simulink model "Planta_6_5_24_V2"  (R2021a)
settings: Solver=VariableStepAuto  StartTime=0.0  StopTime=130  FixedStep=0.002  MaxStep=1e-3  RelTol=1e-4
model workspace (MAT data in the model file):
  VelMin = 0.5
  vMax = -0.3
values from neighbouring files (symbols this model uses):
  ax_max = 0.8    [valoresPlanta_29_9_24.m]    (also in valoresPlanta_v4.m)
  ay_max = 0.75    [valoresPlanta_29_9_24.m]    (also in valoresPlanta_v4.m)
  bcy = 1e7    (= 10000000)    [Valores_1.m]    (also in valoresPlanta.m; valoresPlanta_29_9_24.m; valoresPlanta_V3.m; valoresPlanta_v4.m)
  bh_eq = bhm*ih^2+bhd    (= 8720)    [Valores.m]    (also in Valores_1.m; valoresPlanta.m; valoresPlanta_29_9_24.m; valoresPlanta_V3.m)
  bhb = 1e8    (= 100000000)    [Valores.m]    (also in Valores_1.m; valoresPlanta.m; valoresPlanta_29_9_24.m; valoresPlanta_V3.m)
  bhEb = 2.2e9    (= 2200000000)    [Valores.m]    (also in Valores_1.m; valoresPlanta.m; valoresPlanta_29_9_24.m; valoresPlanta_V3.m)
  bt = 90.0    (= 90)    [Valores.m]    (also in Valores_1.m; valoresPlanta.m; valoresPlanta_29_9_24.m; valoresPlanta_V3.m)
  bt_eq = btd+(btm*(it^2))    (= 5401.8)    [valoresPlanta.m]    (also in valoresPlanta_29_9_24.m; valoresPlanta_V3.m; valoresPlanta_v4.m)
  btb = 5e6    (= 5000000)    [Valores.m]    (also in Valores_1.m; valoresPlanta.m; valoresPlanta_29_9_24.m; valoresPlanta_V3.m)
  btw = 3.0e3    (= 3000)    [Valores.m]    (also in Valores_1.m; valoresPlanta.m; valoresPlanta_29_9_24.m; valoresPlanta_V3.m)
  bwu = 150    [Valores.m]    (also in Valores_1.m; valoresPlanta.m; valoresPlanta_29_9_24.m; valoresPlanta_V3.m)
  estado_cont = [x_positions; hy_cont]    [perfilObsaculos.m]    (also in valoresPlanta_29_9_24.m = [x_positions; [hy_muelle hy_cont]])
  g = 9.80665    [Valores.m]    (also in Valores_1.m; valoresPlanta.m; valoresPlanta_29_9_24.m; valoresPlanta_V3.m)
  Hc = 0    [Valores.m]    (also in Valores_1.m = 2.5; valoresPlanta.m = 2.5; valoresPlanta_29_9_24.m = 2.5; valoresPlanta_V3.m = 2.5)
  hx_cont = 2.5    [perfilObsaculos.m]    (also in puntosTrayectoria.m; valoresPlanta_29_9_24.m)
  ih = 22    [Valores.m]    (also in Valores_1.m; valoresPlanta.m; valoresPlanta_29_9_24.m; valoresPlanta_V3.m)
  it = 30    [Valores.m]    (also in Valores_1.m; valoresPlanta.m; valoresPlanta_29_9_24.m; valoresPlanta_V3.m)
  Jh_eq = Jhm_hb*ih^2+Jhd_hEb    (= 18320)    [Valores.m]    (also in Valores_1.m; valoresPlanta.m; valoresPlanta_29_9_24.m; valoresPlanta_V3.m)
  Jt_eq = Jtd+(Jtm_tb*(it^2))    (= 7500)    [valoresPlanta.m]    (also in valoresPlanta_29_9_24.m; valoresPlanta_V3.m; valoresPlanta_v4.m)
  kcy = 1.8e9    (= 1800000000)    [Valores_1.m]    (also in valoresPlanta.m; valoresPlanta_29_9_24.m; valoresPlanta_V3.m; valoresPlanta_v4.m)
  KDh = Jeq2 * w_posh^3    (= -12245.4404091)    [Valores.m]    (also in Valores_1.m = Jeq2 * w_posh; valoresPlanta.m = Jeq2 * w_posh; valoresPlanta_29_9_24.m = Jh_eq * n * w_posh; valoresPlanta_V3.m = Jeq2 * w_posh)
  KDt = Meq2 * w_post^3    (= -4728.86946035)    [Valores.m]    (also in Valores_1.m = Meq2 * w_post; valoresPlanta.m = Meq2 * w_post; valoresPlanta_29_9_24.m = 10127; valoresPlanta_V3.m = Meq2 * w_post)
  KIh = Jeq2 * w_posh^2    (= 2572.66592082)    [Valores.m]    (also in Valores_1.m = Jeq2 * w_posh^3; valoresPlanta.m = Jeq2 * w_posh^3; valoresPlanta_29_9_24.m = Jh_eq * w_posh^3; valoresPlanta_V3.m = Jeq2 * w_posh^3)
  KIt = Meq2 * w_post^2    (= 1307.690244)    [Valores.m]    (also in Valores_1.m = Meq2 * w_post^3; valoresPlanta.m = Meq2 * w_post^3; valoresPlanta_29_9_24.m = 6809.6; valoresPlanta_V3.m = Meq2 * w_post^3)
  KPh = Jeq2 * w_posh    (= -540.495867769)    [Valores.m]    (also in Valores_1.m = Jeq2 * w_posh^2; valoresPlanta.m = Jeq2 * w_posh^2; valoresPlanta_29_9_24.m = Jh_eq * n * w_posh^2; valoresPlanta_V3.m = Jeq2 * w_posh^2)
  KPt = Meq2 * w_post    (= -361.62)    [Valores.m]    (also in Valores_1.m = Meq2 * w_post^2; valoresPlanta.m = Meq2 * w_post^2; valoresPlanta_29_9_24.m = 14123; valoresPlanta_V3.m = Meq2 * w_post^2)
  Ktw = 4.8e5    (= 480000)    [Valores.m]    (also in Valores_1.m; valoresPlanta.m; valoresPlanta_29_9_24.m; valoresPlanta_V3.m)
  kwu = 2.36e8    (= 236000000)    [Valores.m]    (also in Valores_1.m; valoresPlanta.m; valoresPlanta_29_9_24.m; valoresPlanta_V3.m)
  Mc_max = 5e4    (= 50000)    [Valores.m]    (also in Valores_1.m; valoresPlanta.m; valoresPlanta_29_9_24.m; valoresPlanta_V3.m)
  Mc_min = 2e3    (= 2000)    [Valores.m]    (also in Valores_1.m; valoresPlanta.m; valoresPlanta_29_9_24.m; valoresPlanta_V3.m)
  Meq = Mt+(it^2*Jtm_tb+Jtd)/rtd^2    (= 60000)    [Valores.m]    (also in Valores_1.m; valoresPlanta_29_9_24.m; valoresPlanta_v4.m)
  Ms = 1.5e4    (= 15000)    [Valores.m]    (also in Valores_1.m; valoresPlanta.m; valoresPlanta_29_9_24.m; valoresPlanta_V3.m)
  Mt = 30000    [Valores.m]    (also in Valores_1.m; valoresPlanta.m; valoresPlanta_29_9_24.m; valoresPlanta_V3.m)
  pos = [p0; p1; p2; p3; p4; p5]    [calcularTrayectoria2_prueba.m]    (also in perfilObsaculos.m = puntosTrayectoria(4, 1.5, 20, [-20,0], estado_cont, hy_cont,; puntosTrayectoria.m; valoresPlanta_29_9_24.m = calcularTrayectoria2_prueba(vx_max, vhmax, ax_max, Hc, hx_co)
  rhd = 0.75    [Valores.m]    (also in Valores_1.m; valoresPlanta.m; valoresPlanta_29_9_24.m; valoresPlanta_V3.m)
  rtd = 0.5    [Valores.m]    (also in Valores_1.m; valoresPlanta.m; valoresPlanta_29_9_24.m; valoresPlanta_V3.m)
  tau_hm = 1e-3    (= 0.001)    [valoresPlanta.m]    (also in valoresPlanta_29_9_24.m; valoresPlanta_V3.m; valoresPlanta_v4.m)
  tau_tm = 1e-3    (= 0.001)    [Valores.m]    (also in Valores_1.m; valoresPlanta.m; valoresPlanta_29_9_24.m; valoresPlanta_V3.m)
  Thb_Max = 5e4    (= 50000)    [Valores.m]    (also in Valores_1.m; valoresPlanta.m; valoresPlanta_29_9_24.m; valoresPlanta_V3.m)
  ThEb_Max = 1.1e6    (= 1100000)    [Valores.m]    (also in Valores_1.m; valoresPlanta.m; valoresPlanta_29_9_24.m; valoresPlanta_V3.m)
  Thm_Max = 2e4    (= 20000)    [Valores.m]    (also in Valores_1.m; valoresPlanta.m; valoresPlanta_29_9_24.m; valoresPlanta_V3.m)
  Ttb_Max = 5e3    (= 5000)    [Valores.m]    (also in Valores_1.m; valoresPlanta.m; valoresPlanta_29_9_24.m; valoresPlanta_V3.m)
  Ttm_Max = 3e3    (= 3000)    [Valores.m]    (also in Valores_1.m; valoresPlanta.m; valoresPlanta_29_9_24.m = 4000; valoresPlanta_V3.m)
  vhmax = 3    [valoresPlanta_29_9_24.m]    (also in valoresPlanta_V3.m)
  vx_max = 4    [valoresPlanta_29_9_24.m]
  whmMax = P/Thm_Max    (= 47.8075)    [Valores_1.m]    (also in valoresPlanta.m; valoresPlanta_29_9_24.m = 176; valoresPlanta_V3.m; valoresPlanta_v4.m)
  whmMin = 0.02    [valoresPlanta_29_9_24.m]
  wtmMax = (4/rtd)*it    (= 240)    [Valores_1.m]    (also in valoresPlanta.m; valoresPlanta_29_9_24.m; valoresPlanta_V3.m; valoresPlanta_v4.m)
  wtmMin = 0.02    [valoresPlanta_29_9_24.m]
  x_0 = -20    [valoresPlanta_29_9_24.m]
  x_0_tamb = x_0/rtd    (= -40)    [valoresPlanta_29_9_24.m]
  xLimMax = 49    [valoresPlanta_29_9_24.m]
  xLimMaxSeguridad = 50    [valoresPlanta_29_9_24.m]
  xLimMin = -29    [valoresPlanta_29_9_24.m]
  xLimMinSeguridad = -30    [valoresPlanta_29_9_24.m]
  y_0 = 2.5    [valoresPlanta_29_9_24.m]
  y_0_izaje = 3*(2/rhd)    (= 8)    [valoresPlanta_29_9_24.m]
  yLimMax = 44    [valoresPlanta_29_9_24.m]
  yLimMaxSeguridad = 45    [valoresPlanta_29_9_24.m]
  yLimMin = -19    [valoresPlanta_29_9_24.m]
  yLimMinSeguridad = -20    [valoresPlanta_29_9_24.m]
  Yt0 = 45    [Valores.m]    (also in Valores_1.m; valoresPlanta.m; valoresPlanta_29_9_24.m; valoresPlanta_V3.m)
undefined symbols (not defined in the file or in its folder): DiscIntNeverNeededParam
libraries: simulink x4, vrlib x1, simulink_extras x1, aerolibanimutils x1
(part 3 of 3)

== stateflow chart Planta_6_5_24_V2/Control Supervisor/N_Supervisor ==
  state Nivel_1
    entry:
    estado = 0;
    ml_estimado=0;
    state Movimiento [parallel]
      settings: executionOrder=1
      state Emergencia
        entry:
        vXref = 0;
        vYref = 0;
        %Emergencia = 0;
        %BRKh = 1;
        %BRKt = 1;
      state Manual
        entry:
        ml_estimado = 15000;
        state Movimiento
          entry:
          p0 = [xl, yl]; %Inicial: solo para prueba
          p1 = [x_obj, y_obj]; % p_ref(2,:);
          if (flagSobrecarga == logical(1))
          vYref = min(0, -0.1); % aca usar la velocidad consigna
          vy_max = 0; %v_y_max
          else
          %vYmanualMax = v_y_max;
          %vXmanualMax = vx_max;
          vYref = 0; %v_y_max;
          end
          during:
          p0 = [xl, yl]; %Inicial: solo para prueba
          p1 = [x_obj, y_obj]; % p_ref(2,:);
          %aca actualizar con la consigna
          vYref=vYjoy  ;
          vXref=vXjoy  ;
        state Estimacion_Masa1
          entry:
          vYref = 0.01 * vhmax;
          vXref = 0;
          fhwError= 0.01;
          mMuestras = 4 / 0.02; % muestras en un segundo (20 ms de muestreo)
          [m_temp, fhwEstable] = estimadorMasa(Fhw, fhwError,mMuestras );
          ml_estimado = 15000; %masa del spreader
          m_temp = 0;
          flagFhwEstable = logical(0);
          fhwEstable = logical(0);
          during:
          if (fhwEstable)
          ml_estimado = m_temp;
          fhwEstable = logical(0);
          flagFhwEstable = logical(1);
          else
          [m_temp, fhwEstable] = estimadorMasa(Fhw, fhwError, mMuestras);
          flagFhwEstable = logical(0);
          end
        (default) -> Nivel_1.Movimiento.Manual.Movimiento
        Estimacion_Masa1 -> Nivel_1.Movimiento.Manual.Movimiento : [flagFhwEstable == logical(1)]
        Nivel_1.Movimiento.Manual.Movimiento -> Estimacion_Masa1 [order 2] : [flagCarga || flagDescarga]
      state Inicial
        entry:
        vXref = 0;
        vYref = 0;
        BRKh = 1;
        BRKt = 1;
        % Set de posiciones finales
        p0 = [xl, yl]; %Inicial: solo para prueba
        p1 = [x_obj, y_obj]; % p_ref(2,:);
        during:
        p0 = [xl, yl]; %Inicial: solo para prueba
        p1 = [x_obj, y_obj]; % p_ref(2,:);
        vXref = 0;
        vYref = 0;
        FINISH = 0;
      state estadoVyMax
        entry:
        vy_max = calcVel(ml_estimado, g);
      note: Debe haber un OR para comparar Freno de emergencia y que pase a un estado 0
      state Automatico
        entry:
        FINISH = 0;
        estado = 0;
        %vy_max = calcVel(ml_estimado, g); %cambio ml por ml_estimado
        state perfiles [parallel]
          %entry:
          %v_y_max = calcVel(ml, g);  %MODIFICAR: PONER EN MODO MANUAL
          %v_x_max = vx_max;
          during:
          h_i = pos(1,2);
          h_seg = pos(2,2);
          ds = pos(3,2) - pos(1,2);
          db = pos(4,2) - pos(6,2);
          %y2 = ds - calcPos(ds, v_y_max, ahmax,0);
          %y3 = db - calcPos(db, v_y_max, ahmax,0);
          %funcionaria para 1 ciclo, sino calcular x2 en carro
          %x2 = 10;
          dc = pos(5,1) - pos(2,1);
          %x2 = dc - calcPos(dc, vx_max, ax_max,0);
          settings: executionOrder=1
          state Izaje [parallel]
            settings: executionOrder=2
            state inicial
              entry:
              vYref = 0;
              during:
              vYref = 0;
            state Izaje_subida
              state trayectoria
                entry:
                initialTime_y = currentTime;  %10
                % perfil de velocidad teniendo en cuenta el tiempo, no el espacio a alcanzar
                % totalTime: tiempo necesario para llegar al x final
                PosFinal_y = posicion(3,2)-posicion(1,2);
                %no se si se puede redefinir asi v_max
                [totalTime_y, v_y_max] = calcularTiempoTrapezoidal(PosFinal_y, vy_max, ay_max);
                [vYref, flagFinalizadoY] = generateVelocityProfile(v_y_max, ay_max, currentTime, totalTime_y, initialTime_y);
                during:
                [vYref, flagFinalizadoY] = generateVelocityProfile(v_y_max, ay_max, currentTime, totalTime_y, initialTime_y);
              state detencion
                entry:
                vYref = 0;
                during:
                vYref = 0;
              (default) -> Nivel_1.Movimiento.Automatico.perfiles.Izaje.Izaje_subida.trayectoria
              Nivel_1.Movimiento.Automatico.perfiles.Izaje.Izaje_subida.trayectoria -> Nivel_1.Movimiento.Automatico.perfiles.Izaje.Izaje_subida.detencion : [estado==3]
            state Izaje_bajada
              state trayectoria
                entry:
                initialTime_y = currentTime;  %10
                % perfil de velocidad teniendo en cuenta el tiempo, no el espacio a alcanzar
                % totalTime: tiempo necesario para llegar al x final
                PosFinal_y = abs(posicion(6,2)-posicion(4,2));
                [totalTime_y, v_y_max] = calcularTiempoTrapezoidal(PosFinal_y, vy_max, ay_max);
                [vyref, flagFinalizadoY] = generateVelocityProfile(v_y_max, ay_max, currentTime, totalTime_y, initialTime_y);
                vYref = - vyref;
                during:
                [vyref, flagFinalizadoY] = generateVelocityProfile(v_y_max, ay_max, currentTime, totalTime_y, initialTime_y);
                vYref = - vyref;
              state detencion
                entry:
                vYref = 0;
                during:
                vYref = 0;
              (default) -> Nivel_1.Movimiento.Automatico.perfiles.Izaje.Izaje_bajada.trayectoria
              Nivel_1.Movimiento.Automatico.perfiles.Izaje.Izaje_bajada.trayectoria -> Nivel_1.Movimiento.Automatico.perfiles.Izaje.Izaje_bajada.detencion : [estado==6]
            (default) -> Nivel_1.Movimiento.Automatico.perfiles.Izaje.inicial
            Nivel_1.Movimiento.Automatico.perfiles.Izaje.inicial -> Izaje_subida : [estado == 1]
            Nivel_1.Movimiento.Automatico.perfiles.Izaje.Izaje_subida.detencion -> Izaje_bajada : [estado == 4]
          state Carro_trapezoidal1 [parallel]
            settings: executionOrder=1
            state trayectoria
              entry:
              %v_x_max = vx_max;
              initialTime = currentTime;  %10
              % perfil de velocidad teniendo en cuenta el tiempo, no el espacio a alcanzar
              % totalTime: tiempo necesario para llegar al x final
              PosFinal = posicion(5,1)-posicion(2,1);
              factor = 0;
              if (PosFinal >= 0)
              factor = 1;
              else
              factor = -1;
              end
              [totalTime, v_x_max] = calcularTiempoTrapezoidal(PosFinal, vx_max, ax_max);
              [vxref, flagFinalizadoX] = generateVelocityProfile(v_x_max, ax_max, currentTime, totalTime, initialTime);
              vXref = factor * vxref;
              during:
              [vxref, flagFinalizadoX] = generateVelocityProfile(v_x_max, ax_max, currentTime, totalTime, initialTime);
              vXref = factor * vxref;
            state inicial
              entry:
              vXref = 0;
              during:
              vXref = 0;
            state detencion
              entry:
              vXref = 0;
              during:
              vXref = 0;
            (default) -> Nivel_1.Movimiento.Automatico.perfiles.Carro_trapezoidal1.inicial
            Nivel_1.Movimiento.Automatico.perfiles.Carro_trapezoidal1.inicial -> Nivel_1.Movimiento.Automatico.perfiles.Carro_trapezoidal1.trayectoria : [estado == 2]
            Nivel_1.Movimiento.Automatico.perfiles.Carro_trapezoidal1.trayectoria -> Nivel_1.Movimiento.Automatico.perfiles.Carro_trapezoidal1.detencion : [estado==5]
        state Estados [parallel]
          settings: executionOrder=2
          state e3
            entry:
            estado = 3;
          state e4
            entry:
            estado = 4;
          note: corregir valores limites
          state e2
            entry:
            estado = 2;
          state e5
            entry:
            estado = 5;
          state e1
            entry:
            estado = 1;
          state e6
            entry:
            estado = 6;
            FINISH = 1;
          state e0
            entry:
            estado = 0;
            posicion = calcularTrayectoria2_prueba(vx_max, vy_max, ax_max, Hc, hx_cont, p1, p0, estado_cont);
          e4 -> e5 : [flagFinalizadoX ==1]
          e2 -> e3 : [(flagFinalizadoY == 1)]
          e3 -> e4 : [((xt) >=posicion(4,1))]
          e1 -> e2 : [(yl >=posicion(2,2))]
          e5 -> e6 : [(flagFinalizadoY == 1)]
          e0 -> e1
          (default) -> e0
      Manual -> Emergencia : [Emergencia == 1]
      Automatico -> Emergencia [order 1] : [Emergencia == 1 || P_EH == 1]
      Emergencia -> Inicial : [START == 1 && AUTO == 0 && Emergencia == 0 && P_EH == 0]
      Inicial -> Emergencia [order 2] : [Emergencia == 1]
      Inicial -> Manual [order 1] : [START == 1 && Emergencia==0]
      Nivel_1.Movimiento.Manual.Movimiento -> estadoVyMax [order 1] : [AUTO == 1]
      (default) -> Inicial
      Automatico -> Inicial [order 2] : [FINISH == 1 && AUTO==0]
      estadoVyMax -> Automatico
    state Freno_Operativo [parallel]
      settings: executionOrder=8
      state Enclavamiento_carro [parallel]
        settings: executionOrder=1
        state OFF
          entry:
          BRKt=1;
        state ON
          entry:
          BRKt=0;
        (default) -> Nivel_1.Freno_Operativo.Enclavamiento_carro.OFF
        Nivel_1.Freno_Operativo.Enclavamiento_carro.ON -> Nivel_1.Freno_Operativo.Enclavamiento_carro.OFF : [abs(wtm)>wtmMin || (AUTO==0) || (estado ~= 6)]
        Nivel_1.Freno_Operativo.Enclavamiento_carro.OFF -> Nivel_1.Freno_Operativo.Enclavamiento_carro.ON : [(abs(wtm)<wtmMin) && (estado == 6)&& (AUTO==1) ]
      state Enclavamiento_izaje [parallel]
        settings: executionOrder=2
        state OFF
          entry:
          BRKh=1;
        state ON
          entry:
          BRKh=0;
        (default) -> Nivel_1.Freno_Operativo.Enclavamiento_izaje.OFF
        Nivel_1.Freno_Operativo.Enclavamiento_izaje.ON -> Nivel_1.Freno_Operativo.Enclavamiento_izaje.OFF : [abs(whm)>whmMin || (AUTO==0) || (estado ~= 6)]
        Nivel_1.Freno_Operativo.Enclavamiento_izaje.OFF -> Nivel_1.Freno_Operativo.Enclavamiento_izaje.ON : [(abs(wtm)<wtmMin) && (estado == 6)&&(AUTO==1)]
    note: [eCon ==1 && Select_TLK ==0 && estado==6]
    state Enclavamiento_TLK [parallel]
      settings: executionOrder=3
      state TLC_Activado
        during:
        tw = 1;
      state TLK_Desactivado
        during:
        tw = 0;
      (default) -> TLK_Desactivado
      TLC_Activado -> TLK_Desactivado : [Select_TLK ==0 && estado==6]
      TLK_Desactivado -> TLC_Activado : [Select_TLK == 1]
    state FDC_Carro [parallel]
      settings: executionOrder=4
      state OFF
        entry:
        flagFDCt = 0;
      state ON
        entry:
        flagFDCt = 1;
      (default) -> Nivel_1.FDC_Carro.OFF
      Nivel_1.FDC_Carro.OFF -> Nivel_1.FDC_Carro.ON : [FDCt_d || FDCt_i]
      Nivel_1.FDC_Carro.ON -> Nivel_1.FDC_Carro.OFF : [~FDCt_d && ~FDCt_i]
    state Sobrevelocidad_Izaje [parallel]
      settings: executionOrder=6
      state OFF
        entry:
        Sobrevel_h = 0;
      state ON
        entry:
        Sobrevel_h = 1;
      (default) -> Nivel_1.Sobrevelocidad_Izaje.OFF
      Nivel_1.Sobrevelocidad_Izaje.OFF -> Nivel_1.Sobrevelocidad_Izaje.ON : [abs(whm)>whmMax * 1.15]
      Nivel_1.Sobrevelocidad_Izaje.ON -> Nivel_1.Sobrevelocidad_Izaje.OFF : [abs(whm)<whmMax]
    state Sobrecarga [parallel]
      settings: executionOrder=9
      state ON
        entry:
        flagSobrecarga = logical(1);
      state OFF
        entry:
        flagSobrecarga = logical(0);
      (default) -> Nivel_1.Sobrecarga.OFF
      Nivel_1.Sobrecarga.OFF -> Nivel_1.Sobrecarga.ON : [ml_estimado>  (Mc_max+Ms)]
      Nivel_1.Sobrecarga.ON -> Nivel_1.Sobrecarga.OFF : [ml_estimado< (Mc_max+Ms)]
    note: [eCon == 0 && Select_TLK == 1]
    state Sobrevelocidad_carro [parallel]
      settings: executionOrder=7
      state OFF
        entry:
        Sobrevel_t = 0;
      state ON
        entry:
        Sobrevel_t = 1;%1;
      (default) -> Nivel_1.Sobrevelocidad_carro.OFF
      Nivel_1.Sobrevelocidad_carro.OFF -> Nivel_1.Sobrevelocidad_carro.ON : [abs(whm)>wtmMax]
      Nivel_1.Sobrevelocidad_carro.ON -> Nivel_1.Sobrevelocidad_carro.OFF : [abs(wtm)<wtmMax]
    state FDC_Izaje [parallel]
      settings: executionOrder=5
      state OFF
        entry:
        flagFDCh = 0;
      state ON
        entry:
        flagFDCh = 1;
      (default) -> Nivel_1.FDC_Izaje.OFF
      Nivel_1.FDC_Izaje.OFF -> Nivel_1.FDC_Izaje.ON : [FDCh_min || FDCh_max]
      Nivel_1.FDC_Izaje.ON -> Nivel_1.FDC_Izaje.OFF : [~FDCh_min && ~FDCh_max]
    state Balanceo [parallel]
      settings: executionOrder=2
      state Activado
        entry:
        mBal = 1;
      state Desactivado
        entry:
        mBal = 0;
      (default) -> Desactivado
      Activado -> Desactivado : [bBal == 0]
      Desactivado -> Activado : [bBal == 1]
  data: forceInput function_input; errorThreshold function_input; maxSamples function_input; mass function_output; isStable function_output; Ml function_input; vMaxY function_output; G function_input; DIS function_input; dx function_output; V function_input; A function_input; x0 function_input; v_max function_input; a_max function_input; current_time function_input; total_time function_input; next_velocity function_output; initial_time function_input; flagF function_output; posicion_final function_input; velocidad_maxima function_input; aceleracion_maxima function_input; tiempo function_output; velocidad_corregida function_output; VX_MAX function_input; VY_MAX function_input; AX_MAX function_input; dy function_input; anchoCont function_input; pos_f function_input; POS function_output; pos_i function_input; E_cont function_input; FDCh_min input; FDCh_max input; FDCt_d input; FDCt_i input; vYjoy input; vXjoy input; xl input size=1; flagDescarga input; yl input size=1; v_x_max local double size=1; h_i local size=1; h_seg local size=1; g parameter size=1; xt input size=1; eCon input size=1; pos parameter; db local size=1; ds local size=1; ax_max parameter size=1; dc local size=1; currentTime input size=1; vXref output double size=1; PosFinal local; initialTime local; totalTime local; PosFinal_y local; initialTime_y local; totalTime_y local; vYref output double size=1; ay_max parameter; vx_max parameter; Hc parameter; hx_cont parameter; vhmax parameter; estado_cont parameter; posicion local; START input; p0 local; p1 local; FINISH output size=1; flagFinalizadoY local; flagFinalizadoX local; vyref local; whm input; wtm input; BRKh output size=1; BRKt output size=1; bBal input size=1; mBal output size=1; whmMax parameter size=1; wtmMax parameter size=1; Fhw input size=1; ml_estimado output size=1; fhwError local size=1; mMuestras local; m_temp local double size=1; AUTO input size=1; x_obj input size=1; y_obj input size=1; Select_TLK input; fhwEstable output boolean size=1; flagFhwEstable local; xLimMin parameter; xLimMax parameter; Mc_max parameter; yLimMax parameter; yLimMin parameter; flagFDCh output; flagFDCt output; Emergencia input; Sobrevel_h output; Sobrevel_t output; wtmMin parameter; whmMin parameter; factor local double size=1 =0; vxref local double size=1; P_EH input; tw output double size=1; Ms parameter; flagSobrecarga output; flagCarga input; estado local size=1; v_y_max local size=1; vy_max output
  function [mass, isStable] = estimadorMasa(forceInput, errorThreshold, maxSamples):
    | function [mass, isStable] = estimadorMasa(forceInput, errorThreshold, maxSamples)
    |     persistent forceBuffer;
    |     persistent numSamples;   
    |     % Inicializa las variables persistentes
    |     if isempty(forceBuffer)
    |         forceBuffer = zeros(maxSamples, 1); % Buffer para almacenar las muestras de fuerza
    |         numSamples = 0;
    |         mass_ant=0;
    |     end
    | 
    |     % Tamaño del buffer para calcular la media
    |     bufferSize = length(forceBuffer);
    | 
    |     % Almacena la muestra de fuerza en el buffer
    |     numSamples = numSamples + 1;
    |     forceBuffer(mod(numSamples - 1, bufferSize) + 1) = forceInput;
    | 
    |     % Calcula la media solo cuando el buffer está lleno
    |     if numSamples == maxSamples
    |         forceMean = mean(forceBuffer);
    | 
    |         % Comprueba si la variación porcentual está dentro del umbral de error
    |         isStable = abs((forceInput - forceMean) / forceMean) < errorThreshold;
    | 
    |         % Calcula la masa utilizando la fórmula de tensión (ajusta según tu configuración)
    |         % gravity = 9.81; % aceleración gravitacional
    |         mass = 2 * forceInput / g;  % g es una variable global definida en valoresPlanta_v4
    |         mass_ant=mass;
    | 
    |         % Reinicia el contador y borra los valores del buffer si no es estable
    |         if ~isStable
    |             numSamples = 0;
    |             forceBuffer = zeros(maxSamples, 1);
    |         else
    |             numSamples = 0;
    |             forceBuffer = zeros(maxSamples, 1);
    |         end
    |     else
    |         % Si el buffer no está lleno, simplemente asigna un valor por defecto
    |         isStable = logical(0);
    |         mass = 0; % O cualquier otro valor predeterminado
    |     end
    | end
    | 
    | 
    | % function [mass, isStable] = estimadorMasa(forceInput, errorThreshold, maxSamples)
    | %     persistent forceBuffer;
    | %     persistent numSamples;
    | % 
    | %     % Inicializa las variables persistentes
    | %     if isempty(forceBuffer)
    | %         forceBuffer = zeros(maxSamples, 1); % Buffer para almacenar las muestras de fuerza
    | %         numSamples = 0;
    | %     end
    | % 
    | %     % Tamaño del buffer para calcular la media
    | %     bufferSize = length(forceBuffer);
    | % 
    | %     % Almacena la muestra de fuerza en el buffer
    | %     numSamples = numSamples + 1;
    | %     forceBuffer(mod(numSamples - 1, bufferSize) + 1) = forceInput;
    | % 
    | %     % Calcula la media de todas las muestras de fuerza
    | %     forceMean = mean(forceBuffer(1:min(numSamples, bufferSize)));
    | % 
    | %     % Comprueba si la variacion porcentual está dentro del umbral de error
    | %     isStable = abs((forceInput - forceMean)/forceMean) < errorThreshold;
    | % 
    | %     % Calcula la masa utilizando la fórmula de tensión (ajusta según tu configuración)
    | %     % gravity = 9.81; % aceleración gravitacional
    | %     mass = 2 * forceInput / g;  % g es una variable global definida en valoresPlanta_v4
    | %     
    | %     % Reinicia el contador y borra los valores del buffer si no es estable
    | %     if ~isStable
    | %         numSamples = 0;
    | %         forceBuffer = zeros(maxSamples, 1);
    | %     end
    | % end
    | 
    | 
    | % function [mass, isStable] = estimadorMasa(forceInput, errorThreshold, maxSamples)
    | %     persistent forceBuffer;
    | %     persistent numSamples;
    | % 
    | %     % Initialize persistent variables
    | %     if isempty(forceBuffer)
    | %         forceBuffer = zeros(maxSamples, 1); % Buffer to store force samples
    | %         numSamples = 0;
    | %     end
    | %     % Buffer size for calculating mean
    | %     bufferSize = length(forceBuffer);
    | %     % Store force sample in the buffer
    | %     numSamples = numSamples + 1;
    | %     forceBuffer(mod(numSamples - 1, bufferSize) + 1) = forceInput;
    | %     % Calculate the mean of all force samples
    | %     forceMean = mean(forceBuffer(1:min(numSamples, bufferSize)));
    | %     % Check if the difference is within the error threshold
    | %     isStable = abs(forceInput - forceMean) < errorThreshold;
    | %     % Calculate mass using tension formula (you may need to adjust this based on your setup)
    | %     % gravity = 9.81; % gravitational acceleration
    | %     mass = 2 * forceInput / g;  %g es variable global definida en valoresPlanta_v4
    | % 
    | % end
  function vMaxY = calcVel(Ml, G):
    | function vMaxY = calcVel(Ml, G)
    | %  vMaxY = 956.15e3/((Ml)*G);
    | % Valor de potencia constante a cumplir
    | % Pconst = 65000*9.80665*1.5;
    | Pconst = 956150;  %[W]
    | vMaxY = 1.5;
    | 
    | % Determinacion de velocidad del izaje segun masa de carga
    | if (Ml <= 32500)
    |     vMaxY = 3;
    | 
    | elseif (Ml <65000)
    |     vMaxY = Pconst / (Ml * g);
    | elseif (Ml >= 65000)
    |     vMaxY = 1.5;
    | end
    | 
    | end
  function dx = calcPos(DIS, V, A, x0):
    | function dx = calcPos(DIS, V, A, x0)
    | %12m es la dis minima para desarrollar max velocidad a Amax 
    | % if DIS<12
    | %     dx = DIS - DIS/3;    %3er tercio
    | % else
    | %     dx = v^2/(2*a);    %para izaje 
    | % end
    | dx = x0 + V^2/(2*A);    %para izaje
    | %si DIS < 2*dx ahi divido en 3
    | end
  function [next_velocity, flagF] = generateVelocityProfile(v_max, a_max, current_time, total_time, initial_time):
    | function [next_velocity, flagF] = generateVelocityProfile(v_max, a_max, current_time, total_time, initial_time)
    |     % Parámetros de tiempo
    |     t_acceleration = v_max / a_max;  % Tiempo de aceleración para alcanzar v_max
    |     t_constant = (total_time - 2 * t_acceleration);  % Tiempo en velocidad constante
    |     
    |     % Ajuste el tiempo actual para tener en cuenta el tiempo inicial
    |     current_time_adjusted = current_time - initial_time;
    |     if current_time_adjusted <= 0
    |         next_velocity = 0;
    |         flagF = 0;
    |     elseif current_time_adjusted <= t_acceleration
    |         next_velocity = a_max * current_time_adjusted;
    |         flagF = 0;
    |     elseif current_time_adjusted > t_acceleration && current_time_adjusted < (total_time - t_acceleration)
    |         next_velocity = v_max;
    |         flagF = 0;
    |     else
    |         time_in_deceleration = total_time - current_time_adjusted;
    |         if time_in_deceleration < 0
    |             next_velocity = 0;
    |             flagF = 1;
    |         else
    |             next_velocity = v_max - a_max * (current_time_adjusted - t_acceleration - t_constant);
    |             flagF = 0;
    |         end
    |     end
    | end
    | 
    | % function next_velocity = generateVelocityProfile(v_max, a_max, current_time, total_time)
    | %     % Parámetros de tiempo
    | %     t_acceleration = v_max / a_max;  % Tiempo de aceleración para alcanzar v_max
    | %     t_constant = (total_time - 2 * t_acceleration);  % Tiempo en velocidad constante
    | %     if current_time <= t_acceleration
    | %         next_velocity = a_max * current_time;
    | %     elseif current_time > t_acceleration && current_time < (total_time - t_acceleration)
    | %         next_velocity = v_max;
    | %     else
    | %         time_in_deceleration = total_time - current_time;
    | %         if time_in_deceleration < 0
    | %             next_velocity = 0;
    | %         else
    | %             next_velocity = v_max - a_max * (current_time - t_acceleration - t_constant);
    | %             %tiempo de desaceleracion: tiempo total - tiempo total acel - tiempo cte 
    | %         end
    | %     end
    | % end
  function [tiempo, velocidad_corregida] = calcularTiempoTrapezoidal(posicion_final, velocidad_maxima, aceleracion_maxima):
    | function [tiempo, velocidad_corregida] = calcularTiempoTrapezoidal(posicion_final, velocidad_maxima, aceleracion_maxima)
    |     % Calcula el tiempo necesario para una trayectoria trapezoidal
    |     
    |     % Verifica si la velocidad máxima es alcanzable con la aceleración máxima
    |     tiempo_aceleracion = velocidad_maxima / aceleracion_maxima;
    |     distancia_aceleracion = 0.5 * velocidad_maxima * tiempo_aceleracion;
    |     
    |     % Calcula la distancia total a recorrer
    |     distancia_total = abs(posicion_final);
    |     
    |     if distancia_total <= 2 * distancia_aceleracion
    |         % No se alcanza la velocidad máxima, la aceleración es limitante
    |         % Calcula el tiempo necesario
    | %         tiempo = 2 * sqrt((distancia_total/2) / aceleracion_maxima);
    |         % d = vo * t + 1/2 * a * t^2
    |         t = sqrt(2 * (distancia_total/2) / aceleracion_maxima);
    |         % Calcula la velocidad corregida
    |         % vf = vo + a * t
    | %         velocidad_corregida = sqrt(2 * aceleracion_maxima * distancia_total);
    |         velocidad_corregida = aceleracion_maxima * t;
    |         tiempo = 2 * t;
    |         if (velocidad_corregida > velocidad_maxima)
    |             %perfil trapezoidal -> equidistante
    |             d = distancia_total/3;    
    |             t1 = sqrt((2 * d)/aceleracion_maxima);
    |             % vf = vo + a * t
    |             % velocidad_corregida = aceleracion_maxima * t1;
    |             t2 = d / velocidad_corregida;
    |             tiempo = (2 * t1) + t2;
    |         end
    |         
    |     else
    |         % Se alcanza la velocidad máxima
    |         tiempo_desaceleracion = velocidad_maxima / aceleracion_maxima;
    |         tiempo = tiempo_aceleracion + (distancia_total - 2 * distancia_aceleracion) / velocidad_maxima + tiempo_desaceleracion;
    |         velocidad_corregida = velocidad_maxima;
    |     end
    | end
    | 
    | 
    | 
    | % function [tiempo, VX_MAX] = calcularTiempoTrapezoidal(posicion_final, velocidad_maxima, aceleracion_maxima)
    | % % si la distancia es demasiado pequeña para poder desarrollar la velocidad,
    | % % reducir la velocidad maxima 
    | % % La salida debe ser la velocidad maxima modificada, o la velocidad maxima
    | % 
    | % % Calcula el tiempo necesario para una trayectoria trapezoidal
    | %     
    | %     % Verifica si la velocidad máxima es alcanzable con la aceleración máxima
    | %     tiempo_aceleracion = velocidad_maxima / aceleracion_maxima;
    | %     distancia_aceleracion = 0.5 * velocidad_maxima * tiempo_aceleracion;
    | %     
    | %     % Calcula el tiempo necesario para desacelerar desde la velocidad máxima
    | %     tiempo_desaceleracion = velocidad_maxima / aceleracion_maxima;
    | %     
    | %     % Calcula la distancia total a recorrer
    | %     distancia_total = abs(posicion_final);
    | %     
    | %     if distancia_total <= 2 * distancia_aceleracion
    | %         % No se alcanza la velocidad máxima, la aceleración es limitante
    | %         
    | %         % Se corrige la velocidad, se mantiene la aceleracion maxima
    | %         VX_MAX = sqrt(2 * aceleracion_maxima * distancia_total/2);
    | %         
    | %         % Es correcto?? 
    | %         tiempo = 2 * sqrt((distancia_total / 2) / aceleracion_maxima);
    | %     else
    | %         % Se alcanza la velocidad máxima
    | %         tiempo = tiempo_aceleracion + (distancia_total - 2 * distancia_aceleracion) / velocidad_maxima + tiempo_desaceleracion;
    | %         VX_MAX = velocidad_maxima;
    | %     end
    | % end
  function POS = calcularTrayectoria2_prueba(VX_MAX, VY_MAX, AX_MAX, dy, anchoCont, pos_f, pos_i, E_cont):
    | function POS = calcularTrayectoria2_prueba(VX_MAX, VY_MAX, AX_MAX, dy, anchoCont, pos_f, pos_i, E_cont)
    |  ysb = 15;
    |     % Las dimensiones al concatenar en consigna son de vectores fila
    |     xi = pos_i(1,1);
    |     yi = pos_i(1,2);
    |     xf = pos_f(1,1);
    |     yf = pos_f(1,2);
    | 
    |     %pos_i y pos_f son vectores (x,y)
    |     theta = atan2(VY_MAX,VX_MAX);   %angulo para alcanzar ambas velocidades máximas
    |     dx = (VX_MAX^2)/(2 * AX_MAX)
    | 
    |     if (2 * dx <= (xf-xi))
    |         [hmax, index] = calcularIndice(xi, xf, anchoCont, E_cont);
    |         disp(hmax);
    |         hp = tan(theta) * dx
    |     else 
    |         [hmax, index] = calcularIndice(xi, xf, anchoCont, E_cont); %calcularIndice(xi, xf, anchoCont, to_obj, E_cont
    |         disp(hmax);
    |         VX_MAX = sqrt(2 * AX_MAX * abs((xf-xi)/2))
    |         theta = atan2(VY_MAX,VX_MAX);
    |         dx = (xf-xi)/2;
    |         hp = tan(theta) * dx
    | %     else (dx > (xf-xi)/2)
    | %         [index, hmax] = calcularIndice(xl, anchoCont, to_where, E_cont)
    | %         VX_MAX = sqrt(2 * AX_MAX * (xf-xi)/2);
    | %         theta = atan2(VY_MAX/VX_MAX);
    | %         dx = (xf-xi)/2
    | %         hp = tan(theta) * dx;
    | %     else
    | %         [index, hmax] = calcularIndice(xl, anchoCont, to_where, E_cont)    
    | %         hp = tan(theta) * dx;
    |     end
    | 
    |      
    |     % si hmax es negativo, lo hago ser 15
    |     if (hmax < 0)
    |         hmax = ysb;
    |         % cambiar la altura
    |     elseif (hmax <= yf)
    |         hmax = yf + dy;
    |         
    |     elseif(hmax < p0(2))
    |         if ((p0(2)+ 2 * dy) < 40)
    |             hmax = p0(2)+ dy;   %a criterio, puede ser 2*dy --> ver que cumpla consigna de velocidad
    |                                 % Altura para desarrollar 3 m/s con a = cte
    |         else
    |             hmax = p0(2);
    |         end
    |     end
    |         
    |     hseg = hmax + 2 * dy;  %altura de seguridad
    |     %hseg debe ser < 40:
    |     if ((hmax + 2*dy) >= 40)
    |         h_seg = 40;
    |     else
    |         h_seg = hmax + 2*dy;
    |     end
    | 
    | %     if (p0(2)> hmax)
    | %         if ((p0(2)+ 2 * dy) < 40)
    | %             hmax = p0(2)+ 2 * dy;
    | %         else
    | %             hmax = p0(2);
    | %         end
    | %     end
    |     
    |     p0 = [xi, yi];
    |     p1 = [xi, hmax];    %es muy jugado, puede chocar si la altura max es indice 1
    |     p2 = [(xi+dx), (hseg)];
    |     p3 = [(xf-dx), (hseg)];
    |     p4 = [xf, hmax];    %debe ser mayor a yf
    |     p5 = [xf, yf];
    |     % Corregir: si p0(1) es mas grande que hmax, hmax >= p0(1) (sin pasar limites)
    |     POS = [p0; p1; p2; p3; p4; p5];
    | end
    |     
    |     
    |  
    | function [hmax, index_max] = calcularIndice(xi, xf, anchoCont, E_cont)
    |     % Calcular el índice del valor más alto
    |     % Debe arrancar desde el inicio (-30), no desde el muelle
    |     % indice negativo: solucionado
    |     % 
    |     index = floor((xi) / anchoCont); % extremo: -11 --> 1
    |     % hacer: floor((xi) / anchoCont) + 1 + 12 (para arrancar en 1.25) 
    |     index = index + 12
    |     
    |     index_obj = floor((xf) / anchoCont);
    |     index_obj = index_obj + 12
    |     
    |     % Verificar la dirección --> usar posiciones en coordenadas
    |     if (index_obj > index)
    |         % Calcular la altura máxima para índices menores al calculado
    |         [hmax, index_max] = max(E_cont(2,index:index_obj)) %posible error: indice de subelemento
    |         index_max = index_max + index -1
    |     elseif (index_obj < index)
    |         %comparar posicion objetivo con la inicial
    |         [hmax, index_max] = max(E_cont(2,index_obj:index))
    |         index_max = index_max + index_obj - 1
    |     else
    |         % Otra opción no especificada
    |         hmax = 0;
    |         index_max = 0;
    |         
    |     end
    | 
    | end

== stateflow chart Planta_6_5_24_V2/Chart5 ==
  state START
    entry:
    start=1;
  state STOP
    entry:
    start=0;
  (default) -> STOP
  START -> STOP : [L3==1 ]
  STOP -> START : [L3==1]
  data: L3 input; start output

== stateflow chart Planta_6_5_24_V2/Chart6 ==
  state MODO_DOBLE
    entry:
    modo=1;
  state MODO_SIMPLE
    entry:
    modo=0;
  (default) -> MODO_SIMPLE
  MODO_DOBLE -> MODO_SIMPLE : [R3==1 ]
  MODO_SIMPLE -> MODO_DOBLE : [R3==1]
  data: R3 input; modo output

== stateflow chart Planta_6_5_24_V2/Chart7 ==
  state Sensibilidad
    during:
    if (abs(vy)<=0.05)
    vyOut=0;
    else
    vyOut=vy;
    end
  (default) -> Sensibilidad
  data: vy input; vyOut output

== stateflow chart Planta_6_5_24_V2/Seteo punto de llegada ==
  state Entrada
    entry:
    x=0;
    y=0;
  state Configuracion
    during:
    if(B==1)
    x=x+1/37;
    else
    x=x;
    end
    if(X==1)
    x=x-1/37;
    else
    x=x;
    end
    if(Y==1)
    y=y+1/37;
    else
    y=y;
    end
    if(A==1)
    y=y-1/37;
    else
    y=y;
    end
  state Salida
    entry:
    x=round(x)
    y=round(y)
  (default) -> Entrada
  Entrada -> Configuracion : [start==1]
  Salida -> Configuracion : [start]
  Configuracion -> Salida : [back==1]
  data: back input; start input; y output; x output; A input; Y input; X input; B input

== stateflow chart Planta_6_5_24_V2/Planta/Masa Aleatoria ==
  state Masa
    entry:
    Mcx = fcn(Mc_max, Mc_min);
  state MasaDescargada
    entry:
    Mcx = 0;
  (default) -> MasaDescargada
  MasaDescargada -> Masa : [modo_tw]
  Masa -> MasaDescargada : [~modo_tw]
  data: Mc_MAX function_input; Mc_MIN function_input; ML function_output; Mc_max parameter; Mcx output; Mc_min parameter; modo_tw input
  function ML = fcn(Mc_MAX, Mc_MIN):
    | function ML = fcn(Mc_MAX, Mc_MIN)
    | %Agregar: sobrecarga
    | %if (flag_carga == 1)
    |     ML = Mc_MIN + (Mc_MAX - Mc_MIN)*rand(1);
    |     %ml = Mc_Max + 0.01 * randi([1,15],1) * Mc_Max;
    | %else
    |  %   ML = 0;
    | %end
    | end

== stateflow chart Planta_6_5_24_V2/Chart1 ==
  state Normal
    entry:
    vMin = -0.2*vh_max;
    vMax = 0.2*vh_max;
  state Sobrecarga
    entry:
    vMin = -0.2*vh_max;
    vMax = 0;
  (default) -> Normal
  Sobrecarga -> Normal : [sobreCarga == logical(0)]
  Normal -> Sobrecarga : [sobreCarga == logical(1)]
  data: vh_max parameter; sobreCarga input; vMax output; vMin output

== stateflow chart Planta_6_5_24_V2/Nivel 2/Subsystem1/Chart1 ==
  state Balanceo
    during:
    [KP,KD,KI,WN]=balanceo(Mt,ml,l,g);
    %[KP,KD,KI,WN]=balanceo(ml, Mt, g, l)
  (default) -> Balanceo
  data: mt function_input; Ml function_input; L function_input; G function_input; Kd function_output; Kp function_output; Ki function_output; wn function_output; l input; ml input; KD output; KP output; g parameter; WN output; Mt parameter; KI output
  function [Kd,Kp,Ki, wn]=balanceo(mt,Ml,L,G):
    | function [Kd,Kp,Ki, wn]=balanceo(mt,Ml,L,G)
    | 
    |     z = 0.9;
    |     wn=1*((mt*G)/(L*(mt+Ml)))^(0.5);
    |     Kd=wn^3;
    |     Kp = wn*((2*z+1)*(L-Kd));
    |     Ki = ((mt*G)/((mt+Ml)^2*(L-Kd)))-((wn^2*(2*z+1))/(mt+Ml));
    |     
    |     
    | 
    | end

== stateflow chart Planta_6_5_24_V2/Nivel 2/Subsystem1/Chart2 ==
  state Balanceo
    during:
    [KP,KD,KI,WN]=balanceoPID(Meq, Mt,ml,l,g)
    %[KP,KD,KI,WN]=balanceo(ml, Mt, g, l)
  (default) -> Balanceo
  data: MEQ function_input; mt function_input; Ml function_input; L function_input; G function_input; Kd function_output; Kp function_output; Ki function_output; wn function_output; l input; ml input; KD output; KP output; g parameter; Meq parameter; WN output; Mt parameter; KI output
  function [Kd,Kp,Ki,wn]=balanceoPID(MEQ, mt,Ml,L,G):
    | function [Kd,Kp,Ki,wn]=balanceoPID(MEQ, mt,Ml,L,G)
    |     
    | %     Kd=(1+(L*(mt+Ml)))/(mt+Ml);
    | %     Kp=(2*0.7*wn)/(mt+Ml);
    | %     w=((mt*G/((mt+Ml)*L))^0.5);
    | %     Kd=(mt*G/w^2 + (mt+Ml)*L)/(Ml+mt);
    | %     Kp=2*0.7*(-(mt+Ml)*L/(Ml+mt)+Kd);
    |     
    |     %correccion agustin
    |     %wn=((mt*G)/(L*(mt+Ml)))^(0.5);
    |     %Kd = L - (mt*G)/((mt+Ml)*wn^2);
    |     %Kp = (2*z*wn)/(L-Kd);
    |     %correcion matias
    |     z = 0.7;
    |     wn=((MEQ*G)/(L*(MEQ+Ml)))^(0.5);
    |     wn = 1 * wn; %el mejor: 2
    |     Ki = ((wn^2)*(Meq*L + Ml*(L+Kd)- Kd*mt) - MEQ*G)/(Ml-mt);
    |     Kp = ((2*z*wn)*((MEQ* L) - Ml*(L+Kd)-(Kd*mt)))/(Ml-mt);
    |     Kd = ((-MEQ*G)/(wn^2) +(MEQ+Ml)*L)* 1/(mt+Ml);    %cambiar
    | end
    |  
    | % function [kp,kd,ki,wn] = balanceo(Ml,mt,G,L)
    | %     xita=0.9;%0.7;
    | %     wn=(mt*G/((mt+Ml)*L))^(1/2);
    | %     kd=-(mt*G/((mt+Ml)*(wn^(3))));
    | %     kp=(kd*(2*xita*wn-wn)+l);
    | %     ki=wn^2*(1-xita)*kd;
    | % end
